simulink model "lab_deritative"  (R2024b)
settings: Solver=VariableStepAuto  StartTime=0.0  StopTime=10.0  RelTol=1e-3
libraries: simulink x1
settings Model: Creator=Ahmad  LastModifiedBy=Ahmad

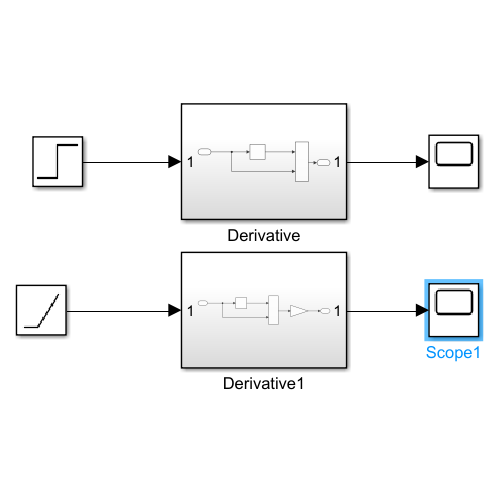
[thumbnail: Simulink's stored preview of the top-level diagram]
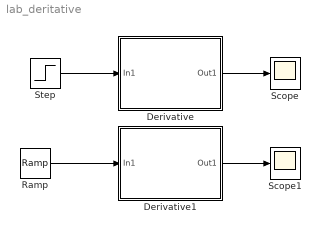
== system lab_deritative ==
  Derivative : Subsystem
  Derivative1 : Subsystem
  Ramp : simulink/Sources/Ramp  slope=1  start=0  InitialOutput=0
  Scope : Scope
  Scope1 : Scope
  Step : Step  SampleTime=0
  wires:
  Step/1 -> Derivative/1(In1)
  Derivative/1(Out1) -> Scope/1
  Derivative1/1(Out1) -> Scope1/1
  Ramp/1 -> Derivative1/1(In1)

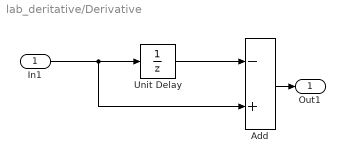
== system lab_deritative/Derivative ==
  In1 : Inport
  Add : Sum  Inputs=-+
  Unit Delay : UnitDelay  SampleTime=-1  HasFrameUpgradeWarning=on
  Out1 : Outport
  wires:
  Add/1 -> Out1/1
  Unit Delay/1 -> Add/1
  In1/1 -> Unit Delay/1, Add/2

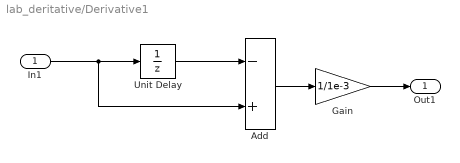
== system lab_deritative/Derivative1 ==
  In1 : Inport
  Add : Sum  Inputs=-+
  Gain : Gain  Gain=1/1e-3
  Unit Delay : UnitDelay  SampleTime=-1  HasFrameUpgradeWarning=on
  Out1 : Outport
  wires:
  Unit Delay/1 -> Add/1
  In1/1 -> Unit Delay/1, Add/2
  Add/1 -> Gain/1
  Gain/1 -> Out1/1
